simulink subsystem "StreetLaneSegment2x1_asSubsystem"  (R2021a)
settings: Solver=VariableStepAuto  StartTime=0.0  StopTime=10.0  RelTol=1e-3
settings Model: Creator=phill  LastModifiedBy=phill

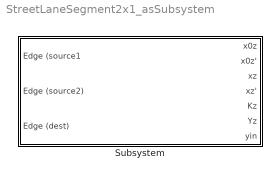
== system StreetLaneSegment2x1_asSubsystem ==
  Subsystem : Subsystem  mask{Kz=0, Tz=0}
      mask prompts: Kz "Kz (Capacity - How many cars fit into this cell)"; Tz "Tz (Nominal travel time for vehicles traveling unobstructed through the cell)"
      mask help: The 2x1 version of the basic 1x1 cell
      mask Display:
      | disp('Street Lane Segment 2x1 \n\n');
      | disp(['Kz = ', get_param(gcb,'Kz'), ' | Tz = ', get_param(gcb, 'Tz')])

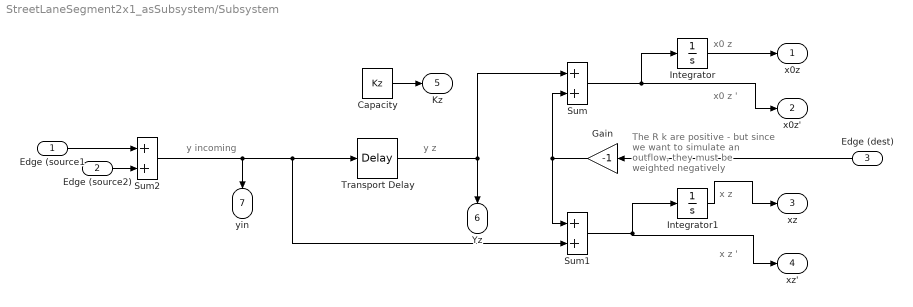
== system StreetLaneSegment2x1_asSubsystem/Subsystem ==
  note: y z
  note: x0 z
  note: y incoming
  note: x z
  note: The R k are positive - but since we
      | want to simulate an outflow, they
      | must be weighted negatively
  note: x z '
  note: x0 z '
  Edge (source1 : Inport
  Edge (source2) : Inport  Port=2
  Edge (dest) : Inport  Port=3
  Capacity : Constant  Value=Kz
  Gain : Gain  Gain=-1
  Integrator : Integrator
  Integrator1 : Integrator
  Sum : Sum
  Sum1 : Sum
  Sum2 : Sum
  Transport Delay : TransportDelay  DelayTime=Tz
  x0z : Outport
  x0z' : Outport  Port=2
  xz : Outport  Port=3
  xz' : Outport  Port=4
  Kz : Outport  Port=5
  Yz : Outport  Port=6
  yin : Outport  Port=7
  wires:
  Transport Delay/1 -> Yz/1, Sum/1
  Sum/1 -> x0z'/1, Integrator/1
  Integrator/1 -> x0z/1
  Capacity/1 -> Kz/1
  Gain/1 -> Sum1/1, Sum/2
  Edge (dest)/1 -> Gain/1
  Sum2/1 -> yin/1, Sum1/2, Transport Delay/1
  Integrator1/1 -> xz/1
  Edge (source2)/1 -> Sum2/2
  Sum1/1 -> xz'/1, Integrator1/1
  Edge (source1/1 -> Sum2/1
